simulink model "question1"  (R2024b)
settings: Solver=VariableStepAuto  StartTime=0.0  StopTime=10.0  RelTol=1e-3
model workspace (MAT data in the model file):
  B = 0.008
  J = 0.093
  Kb = 0.6
  L = 0.006
  R = 0.6
  k = 0.6
settings Model: Creator=Sagar  LastModifiedBy=Sagar

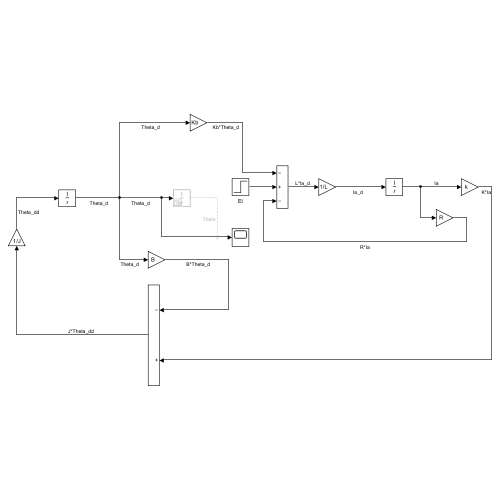
[thumbnail: Simulink's stored preview of the top-level diagram]
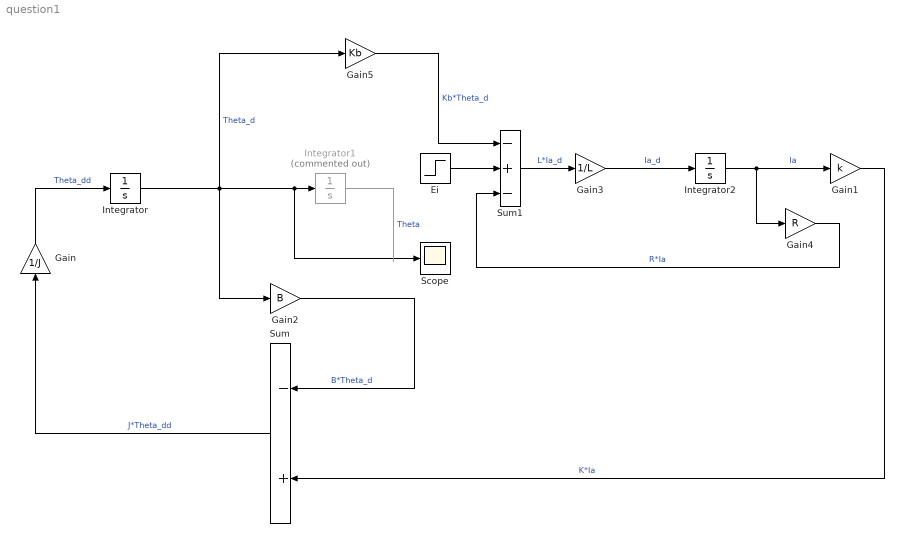
== system question1 ==
  Ei : Step  SampleTime=0
  Gain : Gain  Gain=1/J
  Gain1 : Gain  Gain=k
  Gain2 : Gain  Gain=B
  Gain3 : Gain  Gain=1/L
  Gain4 : Gain  Gain=R
  Gain5 : Gain  Gain=Kb
  Integrator : Integrator
  Integrator1 : Integrator  Commented=on
  Integrator2 : Integrator
  Scope : Scope
  Sum : Sum  Inputs=-+
  Sum1 : Sum  Inputs=-+-
  wires:
  Gain4/1 -> Sum1/3  "R*Ia"
  Integrator/1 -> Gain2/1, Scope/1, Integrator1/1, Gain5/1  "Theta_d"
  Sum1/1 -> Gain3/1  "L*Ia_d"
  Integrator1/1 -> ?  "Theta"
  Gain3/1 -> Integrator2/1  "Ia_d"
  Gain2/1 -> Sum/1  "B*Theta_d"
  Integrator2/1 -> Gain1/1, Gain4/1  "Ia"
  Gain5/1 -> Sum1/1  "Kb*Theta_d"
  Sum/1 -> Gain/1  "J*Theta_dd"
  Gain1/1 -> Sum/2  "K*Ia"
  Gain/1 -> Integrator/1  "Theta_dd"
  Ei/1 -> Sum1/2
